simulink model "node23_case_10kV_withLoad_v2"  (R2022b)
settings: Solver=VariableStepAuto  StartTime=0.0  StopTime=10  FixedStep=1e-6  RelTol=1e-5
InitFcn:
  | sw=5;
  | Lf=1.75e-3+3.5e-3;
  | %Lf=3.5e-3;
  | %Cf=2e-4;
  | f=10;
  | Cf=15e-6;
  | % L=1.75e-3/2;
  | % X=100*pi*L;
  | % R=2*X;
  | R=0.25;X=R/0.66;
  | L=X/100/pi;
  | Z=sqrt(R^2+X^2);
  | f = 30;
  | kp1=10;
  | ki1=100;
  | kp4=20;
  | ki4=100;
  | kp16=20;
  | ki16=100;
  | % 负载参数
  | R1L=0;
  | X1L=0;
  | R2L=652.4467;
  | X2L=276.0351;
  | R3L=804.5741;
  | X3L=256.7790;
  | R4L=760.9867;
  | X4L=234.6376;
  | R5L=818.7384;
  | X5L=266.9799;
  | R6L=671.1329;
  | X6L=170.1801;
  | R7L=883.7621;
  | X7L=178.8663;
  | R8L=388.3725;
  | X8L=158.3040;
  | R9L=817.4819;
  | X9L=268.6933;
  | R10L=849.4733;
  | X10L=254.8420;
  | R11L=407.8415;
  | X11L=165.8504;
  | R12L=NaN;  % Bus 12 无 R、X 数据，用 NaN 标记
  | X12L=NaN;
  | R13L=751.2339;
  | X13L=329.8428;
  | R14L=294.0393;
  | X14L=141.6929;
  | R15L=761.9027;
  | X15L=284.3908;
  | R16L=740.4040;
  | X16L=318.2438;
  | R17L=674.5784;
  | X17L=316.4689;
  | R18L=776.7449;
  | X18L=316.6080;
  | R19L=766.0423;
  | X19L=335.7994;
  | R20L=746.0545;
  | X20L=344.3329;
  | ... (+266 lines)
libraries: spsSeriesRLCBranchLib x210, slpidlib x45, spsControlledVoltageSourceLib x30, spsThreePhaseVIMeasurementLib x24, spsPower3phInstantaneousLib x13, spsAlphaBetaZerotoabcLib x9, spsCurrentMeasurementLib x6, spsGroundLib x2, spspowerguiLib x1
(part 7 of 8)

== system node23_case_10kV_withLoad_v2/IBR-23/SOGI ==
  u : Inport
  Gain1 : Gain  Gain=314.15926
  Gain2 : Gain  Gain=0.707
  Gain3 : Gain  Gain=314.15926
  Integrator : Integrator
  Integrator1 : Integrator
  Sum : Sum  Inputs=-+|
  Sum1 : Sum  Inputs=|+-
  u' : Outport
  qu' : Outport  Port=2
  wires:
  Sum/1 -> Gain2/1
  Gain3/1 -> Sum1/2, qu'/1  "qu'"
  Integrator1/1 -> Gain3/1
  Gain2/1 -> Sum1/1
  Integrator/1 -> Sum/1, u'/1, Integrator1/1  "u'"
  u/1 -> Sum/2
  Sum1/1 -> Gain1/1
  Gain1/1 -> Integrator/1

== system node23_case_10kV_withLoad_v2/IBR-23/k=0.3 ==
  u : Inport
  Gain1 : Gain  Gain=314.15926
  Gain2 : Gain  Gain=0.707
  Gain3 : Gain  Gain=314.15926
  Integrator : Integrator
  Integrator1 : Integrator
  Sum : Sum  Inputs=-+|
  Sum1 : Sum  Inputs=|+-
  u' : Outport
  qu' : Outport  Port=2
  wires:
  Sum/1 -> Gain2/1
  Gain3/1 -> Sum1/2, qu'/1  "qu'"
  Integrator1/1 -> Gain3/1
  Gain2/1 -> Sum1/1
  Integrator/1 -> Sum/1, u'/1, Integrator1/1  "u'"
  u/1 -> Sum/2
  Sum1/1 -> Gain1/1
  Gain1/1 -> Integrator/1

== system node23_case_10kV_withLoad_v2/IBR-8/IBR1输出电压正负序分离 ==
  In1 : Inport
  Add1 : Sum  Inputs=+-
  Add2 : Sum
  Add3 : Sum
  Add4 : Sum  Inputs=+-
  Demux2 : Demux  Outputs=3
  Gain{,1..3} (4 alike) : Gain  Gain=0.5
  Gain4 : Gain  Gain=-1
  abc-alphabeta 1 : MATLAB Function  TreatAsAtomicUnit=on
  albe-dq : MATLAB Function  TreatAsAtomicUnit=on
  alphabeta-dq 1 : MATLAB Function  TreatAsAtomicUnit=on
  k=0.1 : Subsystem
  k=0.4 : Subsystem
  Out1 : Outport  VectorParamsAs1DForOutWhenUnconnected=off
  Out2 : Outport  Port=2  VectorParamsAs1DForOutWhenUnconnected=off
  Out3 : Outport  Port=3  VectorParamsAs1DForOutWhenUnconnected=off
  Out4 : Outport  Port=4  VectorParamsAs1DForOutWhenUnconnected=off
  wires:
  Demux2/2 -> abc-alphabeta 1/2(vb)
  k=0.4/1(u') -> Add3/1, Add1/1
  k=0.1/1(u') -> Add4/1, Add2/2
  Add1/1 -> Gain/1
  Demux2/1 -> abc-alphabeta 1/1(va)
  Gain/1 -> alphabeta-dq 1/1(valpha)
  k=0.4/2(qu') -> Add2/1, Add4/2
  albe-dq/1(vd) -> Out3/1
  k=0.1/2(qu') -> Add1/2, Add3/2
  Add2/1 -> Gain1/1
  alphabeta-dq 1/1(vd) -> Out1/1
  Add3/1 -> Gain2/1
  [wt8] -> Gain4/1
  Gain1/1 -> alphabeta-dq 1/2(vbeta)
  In1/1 -> Demux2/1
  Gain2/1 -> albe-dq/1(valpha)
  alphabeta-dq 1/2(vq) -> Out2/1
  Demux2/3 -> abc-alphabeta 1/3(vc)
  [wt8] -> alphabeta-dq 1/3(ph)
  Gain4/1 -> albe-dq/3(ph)
  albe-dq/2(vq) -> Out4/1
  Add4/1 -> Gain3/1
  abc-alphabeta 1/2(vbeta) -> k=0.1/1(u)
  Gain3/1 -> albe-dq/2(vbeta)
  abc-alphabeta 1/1(valpha) -> k=0.4/1(u)

== system node23_case_10kV_withLoad_v2/IBR-8/IBR1输出电流正负序分离 ==
  In1 : Inport
  Add1 : Sum  Inputs=+-
  Add2 : Sum
  Add3 : Sum
  Add4 : Sum  Inputs=+-
  Demux2 : Demux  Outputs=3
  Gain{,1..3} (4 alike) : Gain  Gain=0.5
  Gain4 : Gain  Gain=-1
  abc-alphabeta 1 : MATLAB Function  TreatAsAtomicUnit=on
  albe-dq : MATLAB Function  TreatAsAtomicUnit=on
  alphabeta-dq 1 : MATLAB Function  TreatAsAtomicUnit=on
  k=0.1 : Subsystem
  k=0.4 : Subsystem
  d+ : Outport  VectorParamsAs1DForOutWhenUnconnected=off
  q+ : Outport  Port=2  VectorParamsAs1DForOutWhenUnconnected=off
  d- : Outport  Port=3  VectorParamsAs1DForOutWhenUnconnected=off
  q- : Outport  Port=4  VectorParamsAs1DForOutWhenUnconnected=off
  wires:
  albe-dq/2(vq) -> q-/1
  albe-dq/1(vd) -> d-/1
  alphabeta-dq 1/2(vq) -> q+/1
  alphabeta-dq 1/1(vd) -> d+/1
  abc-alphabeta 1/1(valpha) -> k=0.4/1(u)
  Gain3/1 -> albe-dq/2(vbeta)
  abc-alphabeta 1/2(vbeta) -> k=0.1/1(u)
  Add4/1 -> Gain3/1
  Gain4/1 -> albe-dq/3(ph)
  [wt8] -> alphabeta-dq 1/3(ph)
  Demux2/3 -> abc-alphabeta 1/3(vc)
  Gain2/1 -> albe-dq/1(valpha)
  In1/1 -> Demux2/1
  Gain1/1 -> alphabeta-dq 1/2(vbeta)
  [wt8] -> Gain4/1
  Add3/1 -> Gain2/1
  Add2/1 -> Gain1/1
  k=0.1/2(qu') -> Add3/2, Add1/2
  k=0.4/2(qu') -> Add4/2, Add2/1
  Gain/1 -> alphabeta-dq 1/1(valpha)
  Demux2/1 -> abc-alphabeta 1/1(va)
  Add1/1 -> Gain/1
  k=0.1/1(u') -> Add2/2, Add4/1
  k=0.4/1(u') -> Add1/1, Add3/1
  Demux2/2 -> abc-alphabeta 1/2(vb)

== system node23_case_10kV_withLoad_v2/IBR-8/SOGI ==
  u : Inport
  Gain1 : Gain  Gain=314.15926
  Gain2 : Gain  Gain=0.707
  Gain3 : Gain  Gain=314.15926
  Integrator : Integrator
  Integrator1 : Integrator
  Sum : Sum  Inputs=-+|
  Sum1 : Sum  Inputs=|+-
  u' : Outport
  qu' : Outport  Port=2
  wires:
  Sum/1 -> Gain2/1
  Gain3/1 -> Sum1/2, qu'/1  "qu'"
  Integrator1/1 -> Gain3/1
  Gain2/1 -> Sum1/1
  Integrator/1 -> Sum/1, u'/1, Integrator1/1  "u'"
  u/1 -> Sum/2
  Sum1/1 -> Gain1/1
  Gain1/1 -> Integrator/1

== system node23_case_10kV_withLoad_v2/IBR-8/k=0.3 ==
  u : Inport
  Gain1 : Gain  Gain=314.15926
  Gain2 : Gain  Gain=0.707
  Gain3 : Gain  Gain=314.15926
  Integrator : Integrator
  Integrator1 : Integrator
  Sum : Sum  Inputs=-+|
  Sum1 : Sum  Inputs=|+-
  u' : Outport
  qu' : Outport  Port=2
  wires:
  Sum/1 -> Gain2/1
  Gain3/1 -> Sum1/2, qu'/1  "qu'"
  Integrator1/1 -> Gain3/1
  Gain2/1 -> Sum1/1
  Integrator/1 -> Sum/1, u'/1, Integrator1/1  "u'"
  u/1 -> Sum/2
  Sum1/1 -> Gain1/1
  Gain1/1 -> Integrator/1

== system node23_case_10kV_withLoad_v2/IBR1输出电压正负序分离/k=0.1 ==
  u : Inport
  Gain1 : Gain  Gain=314.15926
  Gain2 : Gain  Gain=0.707
  Gain3 : Gain  Gain=314.15926
  Integrator : Integrator
  Integrator1 : Integrator
  Sum : Sum  Inputs=-+|
  Sum1 : Sum  Inputs=|+-
  u' : Outport
  qu' : Outport  Port=2
  wires:
  Gain1/1 -> Integrator/1
  Sum1/1 -> Gain1/1
  u/1 -> Sum/2
  Integrator/1 -> Integrator1/1, u'/1, Sum/1  "u'"
  Gain2/1 -> Sum1/1
  Integrator1/1 -> Gain3/1
  Gain3/1 -> qu'/1, Sum1/2  "qu'"
  Sum/1 -> Gain2/1

== system node23_case_10kV_withLoad_v2/IBR1输出电压正负序分离/k=0.4 ==
  u : Inport
  Gain1 : Gain  Gain=314.15926
  Gain2 : Gain  Gain=0.707
  Gain3 : Gain  Gain=314.15926
  Integrator : Integrator
  Integrator1 : Integrator
  Sum : Sum  Inputs=-+|
  Sum1 : Sum  Inputs=|+-
  u' : Outport
  qu' : Outport  Port=2
  wires:
  Gain1/1 -> Integrator/1
  Sum1/1 -> Gain1/1
  u/1 -> Sum/2
  Integrator/1 -> Integrator1/1, u'/1, Sum/1  "u'"
  Gain2/1 -> Sum1/1
  Integrator1/1 -> Gain3/1
  Gain3/1 -> qu'/1, Sum1/2  "qu'"
  Sum/1 -> Gain2/1

== system node23_case_10kV_withLoad_v2/IBR1输出电压正负序分离1/k=0.1 ==
  u : Inport
  Gain1 : Gain  Gain=314.15926
  Gain2 : Gain  Gain=0.707
  Gain3 : Gain  Gain=314.15926
  Integrator : Integrator
  Integrator1 : Integrator
  Sum : Sum  Inputs=-+|
  Sum1 : Sum  Inputs=|+-
  u' : Outport
  qu' : Outport  Port=2
  wires:
  Sum/1 -> Gain2/1
  Gain3/1 -> Sum1/2, qu'/1  "qu'"
  Integrator1/1 -> Gain3/1
  Gain2/1 -> Sum1/1
  Integrator/1 -> Sum/1, u'/1, Integrator1/1  "u'"
  u/1 -> Sum/2
  Sum1/1 -> Gain1/1
  Gain1/1 -> Integrator/1

== system node23_case_10kV_withLoad_v2/IBR1输出电压正负序分离1/k=0.4 ==
  u : Inport
  Gain1 : Gain  Gain=314.15926
  Gain2 : Gain  Gain=0.707
  Gain3 : Gain  Gain=314.15926
  Integrator : Integrator
  Integrator1 : Integrator
  Sum : Sum  Inputs=-+|
  Sum1 : Sum  Inputs=|+-
  u' : Outport
  qu' : Outport  Port=2
  wires:
  Sum/1 -> Gain2/1
  Gain3/1 -> Sum1/2, qu'/1  "qu'"
  Integrator1/1 -> Gain3/1
  Gain2/1 -> Sum1/1
  Integrator/1 -> Sum/1, u'/1, Integrator1/1  "u'"
  u/1 -> Sum/2
  Sum1/1 -> Gain1/1
  Gain1/1 -> Integrator/1

== system node23_case_10kV_withLoad_v2/IBR4/IBR1输出电压正负序分离 ==
  In1 : Inport
  Add1 : Sum  Inputs=+-
  Add2 : Sum
  Add3 : Sum
  Add4 : Sum  Inputs=+-
  Demux2 : Demux  Outputs=3
  Gain{,1..3} (4 alike) : Gain  Gain=0.5
  Gain4 : Gain  Gain=-1
  abc-alphabeta 1 : MATLAB Function  TreatAsAtomicUnit=on
  albe-dq : MATLAB Function  TreatAsAtomicUnit=on
  alphabeta-dq 1 : MATLAB Function  TreatAsAtomicUnit=on
  k=0.1 : Subsystem
  k=0.4 : Subsystem
  vcd_p : Outport  VectorParamsAs1DForOutWhenUnconnected=off
  vcq_p : Outport  Port=2  VectorParamsAs1DForOutWhenUnconnected=off
  vcd_n : Outport  Port=3  VectorParamsAs1DForOutWhenUnconnected=off
  vcq_n : Outport  Port=4  VectorParamsAs1DForOutWhenUnconnected=off
  wires:
  abc-alphabeta 1/1(valpha) -> k=0.4/1(u)
  Gain3/1 -> albe-dq/2(vbeta)
  abc-alphabeta 1/2(vbeta) -> k=0.1/1(u)
  Add4/1 -> Gain3/1
  albe-dq/2(vq) -> vcq_n/1
  Gain4/1 -> albe-dq/3(ph)
  [wt4] -> alphabeta-dq 1/3(ph)
  Demux2/3 -> abc-alphabeta 1/3(vc)
  alphabeta-dq 1/2(vq) -> vcq_p/1
  Gain2/1 -> albe-dq/1(valpha)
  In1/1 -> Demux2/1
  Gain1/1 -> alphabeta-dq 1/2(vbeta)
  [wt4] -> Gain4/1
  Add3/1 -> Gain2/1
  alphabeta-dq 1/1(vd) -> vcd_p/1
  Add2/1 -> Gain1/1
  k=0.1/2(qu') -> Add3/2, Add1/2
  albe-dq/1(vd) -> vcd_n/1
  k=0.4/2(qu') -> Add4/2, Add2/1
  Gain/1 -> alphabeta-dq 1/1(valpha)
  Demux2/1 -> abc-alphabeta 1/1(va)
  Add1/1 -> Gain/1
  k=0.1/1(u') -> Add2/2, Add4/1
  k=0.4/1(u') -> Add1/1, Add3/1
  Demux2/2 -> abc-alphabeta 1/2(vb)

== system node23_case_10kV_withLoad_v2/IBR4/IBR1输出电流正负序分离 ==
  In1 : Inport
  Add1 : Sum  Inputs=+-
  Add2 : Sum
  Add3 : Sum
  Add4 : Sum  Inputs=+-
  Demux2 : Demux  Outputs=3
  Gain{,1..3} (4 alike) : Gain  Gain=0.5
  Gain4 : Gain  Gain=-1
  abc-alphabeta 1 : MATLAB Function  TreatAsAtomicUnit=on
  albe-dq : MATLAB Function  TreatAsAtomicUnit=on
  alphabeta-dq 1 : MATLAB Function  TreatAsAtomicUnit=on
  k=0.1 : Subsystem
  k=0.4 : Subsystem
  d+ : Outport  VectorParamsAs1DForOutWhenUnconnected=off
  q+ : Outport  Port=2  VectorParamsAs1DForOutWhenUnconnected=off
  d- : Outport  Port=3  VectorParamsAs1DForOutWhenUnconnected=off
  q- : Outport  Port=4  VectorParamsAs1DForOutWhenUnconnected=off
  wires:
  Demux2/2 -> abc-alphabeta 1/2(vb)
  k=0.4/1(u') -> Add3/1, Add1/1
  k=0.1/1(u') -> Add4/1, Add2/2
  Add1/1 -> Gain/1
  Demux2/1 -> abc-alphabeta 1/1(va)
  Gain/1 -> alphabeta-dq 1/1(valpha)
  k=0.4/2(qu') -> Add2/1, Add4/2
  k=0.1/2(qu') -> Add1/2, Add3/2
  Add2/1 -> Gain1/1
  Add3/1 -> Gain2/1
  [wt4] -> Gain4/1
  Gain1/1 -> alphabeta-dq 1/2(vbeta)
  In1/1 -> Demux2/1
  Gain2/1 -> albe-dq/1(valpha)
  Demux2/3 -> abc-alphabeta 1/3(vc)
  [wt4] -> alphabeta-dq 1/3(ph)
  Gain4/1 -> albe-dq/3(ph)
  Add4/1 -> Gain3/1
  abc-alphabeta 1/2(vbeta) -> k=0.1/1(u)
  Gain3/1 -> albe-dq/2(vbeta)
  abc-alphabeta 1/1(valpha) -> k=0.4/1(u)
  alphabeta-dq 1/1(vd) -> d+/1
  alphabeta-dq 1/2(vq) -> q+/1
  albe-dq/1(vd) -> d-/1
  albe-dq/2(vq) -> q-/1

== system node23_case_10kV_withLoad_v2/IBR4/SOGI ==
  u : Inport
  Gain1 : Gain  Gain=314.15926
  Gain2 : Gain  Gain=0.707
  Gain3 : Gain  Gain=314.15926
  Integrator : Integrator
  Integrator1 : Integrator
  Sum : Sum  Inputs=-+|
  Sum1 : Sum  Inputs=|+-
  u' : Outport
  qu' : Outport  Port=2
  wires:
  Sum/1 -> Gain2/1
  Gain3/1 -> Sum1/2, qu'/1  "qu'"
  Integrator1/1 -> Gain3/1
  Gain2/1 -> Sum1/1
  Integrator/1 -> Sum/1, u'/1, Integrator1/1  "u'"
  u/1 -> Sum/2
  Sum1/1 -> Gain1/1
  Gain1/1 -> Integrator/1

== system node23_case_10kV_withLoad_v2/IBR4/k=0.3 ==
  u : Inport
  Gain1 : Gain  Gain=314.15926
  Gain2 : Gain  Gain=0.707
  Gain3 : Gain  Gain=314.15926
  Integrator : Integrator
  Integrator1 : Integrator
  Sum : Sum  Inputs=-+|
  Sum1 : Sum  Inputs=|+-
  u' : Outport
  qu' : Outport  Port=2
  wires:
  Sum/1 -> Gain2/1
  Gain3/1 -> Sum1/2, qu'/1  "qu'"
  Integrator1/1 -> Gain3/1
  Gain2/1 -> Sum1/1
  Integrator/1 -> Sum/1, u'/1, Integrator1/1  "u'"
  u/1 -> Sum/2
  Sum1/1 -> Gain1/1
  Gain1/1 -> Integrator/1

== system node23_case_10kV_withLoad_v2/电网电压正负序分离/k=0.1 ==
  u : Inport
  Gain1 : Gain  Gain=314.15926
  Gain2 : Gain  Gain=0.707
  Gain3 : Gain  Gain=314.15926
  Integrator : Integrator
  Integrator1 : Integrator
  Sum : Sum  Inputs=-+|
  Sum1 : Sum  Inputs=|+-
  u' : Outport
  qu' : Outport  Port=2
  wires:
  Gain1/1 -> Integrator/1
  Sum1/1 -> Gain1/1
  u/1 -> Sum/2
  Integrator/1 -> Integrator1/1, u'/1, Sum/1  "u'"
  Gain2/1 -> Sum1/1
  Integrator1/1 -> Gain3/1
  Gain3/1 -> qu'/1, Sum1/2  "qu'"
  Sum/1 -> Gain2/1

== system node23_case_10kV_withLoad_v2/电网电压正负序分离/k=0.4 ==
  u : Inport
  Gain1 : Gain  Gain=314.15926
  Gain2 : Gain  Gain=0.707
  Gain3 : Gain  Gain=314.15926
  Integrator : Integrator
  Integrator1 : Integrator
  Sum : Sum  Inputs=-+|
  Sum1 : Sum  Inputs=|+-
  u' : Outport
  qu' : Outport  Port=2
  wires:
  Gain1/1 -> Integrator/1
  Sum1/1 -> Gain1/1
  u/1 -> Sum/2
  Integrator/1 -> Integrator1/1, u'/1, Sum/1  "u'"
  Gain2/1 -> Sum1/1
  Integrator1/1 -> Gain3/1
  Gain3/1 -> qu'/1, Sum1/2  "qu'"
  Sum/1 -> Gain2/1

== system node23_case_10kV_withLoad_v2/Grid/negative_sequence_dq>>abc4/dq0>>alpha_beta_0 ==
  alpha_beta_0 : Inport
  Gain3 : Gain  Gain="[ 1   0   1; -1/2  sqrt(3)/2   1; -1/2  -sqrt(3)/2  1 ]"  Multiplication=Matrix(K*u) (u vector)  SaturateOnIntegerOverflow=on  OutDataTypeStr=Inherit: Same as input  ParamDataTypeStr=Inherit: Same as input
  abc : Outport
  wires:
  alpha_beta_0/1 -> Gain3/1
  Gain3/1 -> abc/1

== system node23_case_10kV_withLoad_v2/Grid/positive_sequence_dq>>abc1/dq0>>alpha_beta_0 ==
  alpha_beta_0 : Inport
  Gain3 : Gain  Gain="[ 1   0   1; -1/2  sqrt(3)/2   1; -1/2  -sqrt(3)/2  1 ]"  Multiplication=Matrix(K*u) (u vector)  SaturateOnIntegerOverflow=on  OutDataTypeStr=Inherit: Same as input  ParamDataTypeStr=Inherit: Same as input
  abc : Outport
  wires:
  alpha_beta_0/1 -> Gain3/1
  Gain3/1 -> abc/1

== system node23_case_10kV_withLoad_v2/IBR-10/IBR1输出电压正负序分离/k=0.1 ==
  u : Inport
  Gain1 : Gain  Gain=314.15926
  Gain2 : Gain  Gain=0.707
  Gain3 : Gain  Gain=314.15926
  Integrator : Integrator
  Integrator1 : Integrator
  Sum : Sum  Inputs=-+|
  Sum1 : Sum  Inputs=|+-
  u' : Outport
  qu' : Outport  Port=2
  wires:
  Sum/1 -> Gain2/1
  Gain3/1 -> Sum1/2, qu'/1  "qu'"
  Integrator1/1 -> Gain3/1
  Gain2/1 -> Sum1/1
  Integrator/1 -> Sum/1, u'/1, Integrator1/1  "u'"
  u/1 -> Sum/2
  Sum1/1 -> Gain1/1
  Gain1/1 -> Integrator/1

== system node23_case_10kV_withLoad_v2/IBR-10/IBR1输出电压正负序分离/k=0.4 ==
  u : Inport
  Gain1 : Gain  Gain=314.15926
  Gain2 : Gain  Gain=0.707
  Gain3 : Gain  Gain=314.15926
  Integrator : Integrator
  Integrator1 : Integrator
  Sum : Sum  Inputs=-+|
  Sum1 : Sum  Inputs=|+-
  u' : Outport
  qu' : Outport  Port=2
  wires:
  Sum/1 -> Gain2/1
  Gain3/1 -> Sum1/2, qu'/1  "qu'"
  Integrator1/1 -> Gain3/1
  Gain2/1 -> Sum1/1
  Integrator/1 -> Sum/1, u'/1, Integrator1/1  "u'"
  u/1 -> Sum/2
  Sum1/1 -> Gain1/1
  Gain1/1 -> Integrator/1

== system node23_case_10kV_withLoad_v2/IBR-10/IBR1输出电流正负序分离/k=0.1 ==
  u : Inport
  Gain1 : Gain  Gain=314.15926
  Gain2 : Gain  Gain=0.707
  Gain3 : Gain  Gain=314.15926
  Integrator : Integrator
  Integrator1 : Integrator
  Sum : Sum  Inputs=-+|
  Sum1 : Sum  Inputs=|+-
  u' : Outport
  qu' : Outport  Port=2
  wires:
  Gain1/1 -> Integrator/1
  Sum1/1 -> Gain1/1
  u/1 -> Sum/2
  Integrator/1 -> Integrator1/1, u'/1, Sum/1  "u'"
  Gain2/1 -> Sum1/1
  Integrator1/1 -> Gain3/1
  Gain3/1 -> qu'/1, Sum1/2  "qu'"
  Sum/1 -> Gain2/1

== system node23_case_10kV_withLoad_v2/IBR-10/IBR1输出电流正负序分离/k=0.4 ==
  u : Inport
  Gain1 : Gain  Gain=314.15926
  Gain2 : Gain  Gain=0.707
  Gain3 : Gain  Gain=314.15926
  Integrator : Integrator
  Integrator1 : Integrator
  Sum : Sum  Inputs=-+|
  Sum1 : Sum  Inputs=|+-
  u' : Outport
  qu' : Outport  Port=2
  wires:
  Gain1/1 -> Integrator/1
  Sum1/1 -> Gain1/1
  u/1 -> Sum/2
  Integrator/1 -> Integrator1/1, u'/1, Sum/1  "u'"
  Gain2/1 -> Sum1/1
  Integrator1/1 -> Gain3/1
  Gain3/1 -> qu'/1, Sum1/2  "qu'"
  Sum/1 -> Gain2/1

== system node23_case_10kV_withLoad_v2/IBR-11/IBR1输出电压正负序分离/k=0.1 ==
  u : Inport
  Gain1 : Gain  Gain=314.15926
  Gain2 : Gain  Gain=0.707
  Gain3 : Gain  Gain=314.15926
  Integrator : Integrator
  Integrator1 : Integrator
  Sum : Sum  Inputs=-+|
  Sum1 : Sum  Inputs=|+-
  u' : Outport
  qu' : Outport  Port=2
  wires:
  Sum/1 -> Gain2/1
  Gain3/1 -> Sum1/2, qu'/1  "qu'"
  Integrator1/1 -> Gain3/1
  Gain2/1 -> Sum1/1
  Integrator/1 -> Sum/1, u'/1, Integrator1/1  "u'"
  u/1 -> Sum/2
  Sum1/1 -> Gain1/1
  Gain1/1 -> Integrator/1

== system node23_case_10kV_withLoad_v2/IBR-11/IBR1输出电压正负序分离/k=0.4 ==
  u : Inport
  Gain1 : Gain  Gain=314.15926
  Gain2 : Gain  Gain=0.707
  Gain3 : Gain  Gain=314.15926
  Integrator : Integrator
  Integrator1 : Integrator
  Sum : Sum  Inputs=-+|
  Sum1 : Sum  Inputs=|+-
  u' : Outport
  qu' : Outport  Port=2
  wires:
  Sum/1 -> Gain2/1
  Gain3/1 -> Sum1/2, qu'/1  "qu'"
  Integrator1/1 -> Gain3/1
  Gain2/1 -> Sum1/1
  Integrator/1 -> Sum/1, u'/1, Integrator1/1  "u'"
  u/1 -> Sum/2
  Sum1/1 -> Gain1/1
  Gain1/1 -> Integrator/1

== system node23_case_10kV_withLoad_v2/IBR-11/IBR1输出电流正负序分离/k=0.1 ==
  u : Inport
  Gain1 : Gain  Gain=314.15926
  Gain2 : Gain  Gain=0.707
  Gain3 : Gain  Gain=314.15926
  Integrator : Integrator
  Integrator1 : Integrator
  Sum : Sum  Inputs=-+|
  Sum1 : Sum  Inputs=|+-
  u' : Outport
  qu' : Outport  Port=2
  wires:
  Gain1/1 -> Integrator/1
  Sum1/1 -> Gain1/1
  u/1 -> Sum/2
  Integrator/1 -> Integrator1/1, u'/1, Sum/1  "u'"
  Gain2/1 -> Sum1/1
  Integrator1/1 -> Gain3/1
  Gain3/1 -> qu'/1, Sum1/2  "qu'"
  Sum/1 -> Gain2/1

== system node23_case_10kV_withLoad_v2/IBR-11/IBR1输出电流正负序分离/k=0.4 ==
  u : Inport
  Gain1 : Gain  Gain=314.15926
  Gain2 : Gain  Gain=0.707
  Gain3 : Gain  Gain=314.15926
  Integrator : Integrator
  Integrator1 : Integrator
  Sum : Sum  Inputs=-+|
  Sum1 : Sum  Inputs=|+-
  u' : Outport
  qu' : Outport  Port=2
  wires:
  Gain1/1 -> Integrator/1
  Sum1/1 -> Gain1/1
  u/1 -> Sum/2
  Integrator/1 -> Integrator1/1, u'/1, Sum/1  "u'"
  Gain2/1 -> Sum1/1
  Integrator1/1 -> Gain3/1
  Gain3/1 -> qu'/1, Sum1/2  "qu'"
  Sum/1 -> Gain2/1

== system node23_case_10kV_withLoad_v2/IBR-12/IBR1输出电压正负序分离/k=0.1 ==
  u : Inport
  Gain1 : Gain  Gain=314.15926
  Gain2 : Gain  Gain=0.707
  Gain3 : Gain  Gain=314.15926
  Integrator : Integrator
  Integrator1 : Integrator
  Sum : Sum  Inputs=-+|
  Sum1 : Sum  Inputs=|+-
  u' : Outport
  qu' : Outport  Port=2
  wires:
  Sum/1 -> Gain2/1
  Gain3/1 -> Sum1/2, qu'/1  "qu'"
  Integrator1/1 -> Gain3/1
  Gain2/1 -> Sum1/1
  Integrator/1 -> Sum/1, u'/1, Integrator1/1  "u'"
  u/1 -> Sum/2
  Sum1/1 -> Gain1/1
  Gain1/1 -> Integrator/1

== system node23_case_10kV_withLoad_v2/IBR-12/IBR1输出电压正负序分离/k=0.4 ==
  u : Inport
  Gain1 : Gain  Gain=314.15926
  Gain2 : Gain  Gain=0.707
  Gain3 : Gain  Gain=314.15926
  Integrator : Integrator
  Integrator1 : Integrator
  Sum : Sum  Inputs=-+|
  Sum1 : Sum  Inputs=|+-
  u' : Outport
  qu' : Outport  Port=2
  wires:
  Sum/1 -> Gain2/1
  Gain3/1 -> Sum1/2, qu'/1  "qu'"
  Integrator1/1 -> Gain3/1
  Gain2/1 -> Sum1/1
  Integrator/1 -> Sum/1, u'/1, Integrator1/1  "u'"
  u/1 -> Sum/2
  Sum1/1 -> Gain1/1
  Gain1/1 -> Integrator/1

== system node23_case_10kV_withLoad_v2/IBR-12/IBR1输出电流正负序分离/k=0.1 ==
  u : Inport
  Gain1 : Gain  Gain=314.15926
  Gain2 : Gain  Gain=0.707
  Gain3 : Gain  Gain=314.15926
  Integrator : Integrator
  Integrator1 : Integrator
  Sum : Sum  Inputs=-+|
  Sum1 : Sum  Inputs=|+-
  u' : Outport
  qu' : Outport  Port=2
  wires:
  Gain1/1 -> Integrator/1
  Sum1/1 -> Gain1/1
  u/1 -> Sum/2
  Integrator/1 -> Integrator1/1, u'/1, Sum/1  "u'"
  Gain2/1 -> Sum1/1
  Integrator1/1 -> Gain3/1
  Gain3/1 -> qu'/1, Sum1/2  "qu'"
  Sum/1 -> Gain2/1

== system node23_case_10kV_withLoad_v2/IBR-12/IBR1输出电流正负序分离/k=0.4 ==
  u : Inport
  Gain1 : Gain  Gain=314.15926
  Gain2 : Gain  Gain=0.707
  Gain3 : Gain  Gain=314.15926
  Integrator : Integrator
  Integrator1 : Integrator
  Sum : Sum  Inputs=-+|
  Sum1 : Sum  Inputs=|+-
  u' : Outport
  qu' : Outport  Port=2
  wires:
  Gain1/1 -> Integrator/1
  Sum1/1 -> Gain1/1
  u/1 -> Sum/2
  Integrator/1 -> Integrator1/1, u'/1, Sum/1  "u'"
  Gain2/1 -> Sum1/1
  Integrator1/1 -> Gain3/1
  Gain3/1 -> qu'/1, Sum1/2  "qu'"
  Sum/1 -> Gain2/1

== system node23_case_10kV_withLoad_v2/IBR-16/IBR1输出电压正负序分离/k=0.1 ==
  u : Inport
  Gain1 : Gain  Gain=314.15926
  Gain2 : Gain  Gain=0.707
  Gain3 : Gain  Gain=314.15926
  Integrator : Integrator
  Integrator1 : Integrator
  Sum : Sum  Inputs=-+|
  Sum1 : Sum  Inputs=|+-
  u' : Outport
  qu' : Outport  Port=2
  wires:
  Sum/1 -> Gain2/1
  Gain3/1 -> Sum1/2, qu'/1  "qu'"
  Integrator1/1 -> Gain3/1
  Gain2/1 -> Sum1/1
  Integrator/1 -> Sum/1, u'/1, Integrator1/1  "u'"
  u/1 -> Sum/2
  Sum1/1 -> Gain1/1
  Gain1/1 -> Integrator/1

== system node23_case_10kV_withLoad_v2/IBR-16/IBR1输出电压正负序分离/k=0.4 ==
  u : Inport
  Gain1 : Gain  Gain=314.15926
  Gain2 : Gain  Gain=0.707
  Gain3 : Gain  Gain=314.15926
  Integrator : Integrator
  Integrator1 : Integrator
  Sum : Sum  Inputs=-+|
  Sum1 : Sum  Inputs=|+-
  u' : Outport
  qu' : Outport  Port=2
  wires:
  Sum/1 -> Gain2/1
  Gain3/1 -> Sum1/2, qu'/1  "qu'"
  Integrator1/1 -> Gain3/1
  Gain2/1 -> Sum1/1
  Integrator/1 -> Sum/1, u'/1, Integrator1/1  "u'"
  u/1 -> Sum/2
  Sum1/1 -> Gain1/1
  Gain1/1 -> Integrator/1

== system node23_case_10kV_withLoad_v2/IBR-16/IBR1输出电流正负序分离/k=0.1 ==
  u : Inport
  Gain1 : Gain  Gain=314.15926
  Gain2 : Gain  Gain=0.707
  Gain3 : Gain  Gain=314.15926
  Integrator : Integrator
  Integrator1 : Integrator
  Sum : Sum  Inputs=-+|
  Sum1 : Sum  Inputs=|+-
  u' : Outport
  qu' : Outport  Port=2
  wires:
  Gain1/1 -> Integrator/1
  Sum1/1 -> Gain1/1
  u/1 -> Sum/2
  Integrator/1 -> Integrator1/1, u'/1, Sum/1  "u'"
  Gain2/1 -> Sum1/1
  Integrator1/1 -> Gain3/1
  Gain3/1 -> qu'/1, Sum1/2  "qu'"
  Sum/1 -> Gain2/1

== system node23_case_10kV_withLoad_v2/IBR-16/IBR1输出电流正负序分离/k=0.4 ==
  u : Inport
  Gain1 : Gain  Gain=314.15926
  Gain2 : Gain  Gain=0.707
  Gain3 : Gain  Gain=314.15926
  Integrator : Integrator
  Integrator1 : Integrator
  Sum : Sum  Inputs=-+|
  Sum1 : Sum  Inputs=|+-
  u' : Outport
  qu' : Outport  Port=2
  wires:
  Gain1/1 -> Integrator/1
  Sum1/1 -> Gain1/1
  u/1 -> Sum/2
  Integrator/1 -> Integrator1/1, u'/1, Sum/1  "u'"
  Gain2/1 -> Sum1/1
  Integrator1/1 -> Gain3/1
  Gain3/1 -> qu'/1, Sum1/2  "qu'"
  Sum/1 -> Gain2/1

== system node23_case_10kV_withLoad_v2/IBR-21/IBR1输出电压正负序分离/k=0.1 ==
  u : Inport
  Gain1 : Gain  Gain=314.15926
  Gain2 : Gain  Gain=0.707
  Gain3 : Gain  Gain=314.15926
  Integrator : Integrator
  Integrator1 : Integrator
  Sum : Sum  Inputs=-+|
  Sum1 : Sum  Inputs=|+-
  u' : Outport
  qu' : Outport  Port=2
  wires:
  Sum/1 -> Gain2/1
  Gain3/1 -> Sum1/2, qu'/1  "qu'"
  Integrator1/1 -> Gain3/1
  Gain2/1 -> Sum1/1
  Integrator/1 -> Sum/1, u'/1, Integrator1/1  "u'"
  u/1 -> Sum/2
  Sum1/1 -> Gain1/1
  Gain1/1 -> Integrator/1

== system node23_case_10kV_withLoad_v2/IBR-21/IBR1输出电压正负序分离/k=0.4 ==
  u : Inport
  Gain1 : Gain  Gain=314.15926
  Gain2 : Gain  Gain=0.707
  Gain3 : Gain  Gain=314.15926
  Integrator : Integrator
  Integrator1 : Integrator
  Sum : Sum  Inputs=-+|
  Sum1 : Sum  Inputs=|+-
  u' : Outport
  qu' : Outport  Port=2
  wires:
  Sum/1 -> Gain2/1
  Gain3/1 -> Sum1/2, qu'/1  "qu'"
  Integrator1/1 -> Gain3/1
  Gain2/1 -> Sum1/1
  Integrator/1 -> Sum/1, u'/1, Integrator1/1  "u'"
  u/1 -> Sum/2
  Sum1/1 -> Gain1/1
  Gain1/1 -> Integrator/1

== system node23_case_10kV_withLoad_v2/IBR-21/IBR1输出电流正负序分离/k=0.1 ==
  u : Inport
  Gain1 : Gain  Gain=314.15926
  Gain2 : Gain  Gain=0.707
  Gain3 : Gain  Gain=314.15926
  Integrator : Integrator
  Integrator1 : Integrator
  Sum : Sum  Inputs=-+|
  Sum1 : Sum  Inputs=|+-
  u' : Outport
  qu' : Outport  Port=2
  wires:
  Gain1/1 -> Integrator/1
  Sum1/1 -> Gain1/1
  u/1 -> Sum/2
  Integrator/1 -> Integrator1/1, u'/1, Sum/1  "u'"
  Gain2/1 -> Sum1/1
  Integrator1/1 -> Gain3/1
  Gain3/1 -> qu'/1, Sum1/2  "qu'"
  Sum/1 -> Gain2/1

== system node23_case_10kV_withLoad_v2/IBR-21/IBR1输出电流正负序分离/k=0.4 ==
  u : Inport
  Gain1 : Gain  Gain=314.15926
  Gain2 : Gain  Gain=0.707
  Gain3 : Gain  Gain=314.15926
  Integrator : Integrator
  Integrator1 : Integrator
  Sum : Sum  Inputs=-+|
  Sum1 : Sum  Inputs=|+-
  u' : Outport
  qu' : Outport  Port=2
  wires:
  Gain1/1 -> Integrator/1
  Sum1/1 -> Gain1/1
  u/1 -> Sum/2
  Integrator/1 -> Integrator1/1, u'/1, Sum/1  "u'"
  Gain2/1 -> Sum1/1
  Integrator1/1 -> Gain3/1
  Gain3/1 -> qu'/1, Sum1/2  "qu'"
  Sum/1 -> Gain2/1

== system node23_case_10kV_withLoad_v2/IBR-22/IBR1输出电压正负序分离/k=0.1 ==
  u : Inport
  Gain1 : Gain  Gain=314.15926
  Gain2 : Gain  Gain=0.707
  Gain3 : Gain  Gain=314.15926
  Integrator : Integrator
  Integrator1 : Integrator
  Sum : Sum  Inputs=-+|
  Sum1 : Sum  Inputs=|+-
  u' : Outport
  qu' : Outport  Port=2
  wires:
  Sum/1 -> Gain2/1
  Gain3/1 -> Sum1/2, qu'/1  "qu'"
  Integrator1/1 -> Gain3/1
  Gain2/1 -> Sum1/1
  Integrator/1 -> Sum/1, u'/1, Integrator1/1  "u'"
  u/1 -> Sum/2
  Sum1/1 -> Gain1/1
  Gain1/1 -> Integrator/1

== system node23_case_10kV_withLoad_v2/IBR-22/IBR1输出电压正负序分离/k=0.4 ==
  u : Inport
  Gain1 : Gain  Gain=314.15926
  Gain2 : Gain  Gain=0.707
  Gain3 : Gain  Gain=314.15926
  Integrator : Integrator
  Integrator1 : Integrator
  Sum : Sum  Inputs=-+|
  Sum1 : Sum  Inputs=|+-
  u' : Outport
  qu' : Outport  Port=2
  wires:
  Sum/1 -> Gain2/1
  Gain3/1 -> Sum1/2, qu'/1  "qu'"
  Integrator1/1 -> Gain3/1
  Gain2/1 -> Sum1/1
  Integrator/1 -> Sum/1, u'/1, Integrator1/1  "u'"
  u/1 -> Sum/2
  Sum1/1 -> Gain1/1
  Gain1/1 -> Integrator/1

== system node23_case_10kV_withLoad_v2/IBR-22/IBR1输出电流正负序分离/k=0.1 ==
  u : Inport
  Gain1 : Gain  Gain=314.15926
  Gain2 : Gain  Gain=0.707
  Gain3 : Gain  Gain=314.15926
  Integrator : Integrator
  Integrator1 : Integrator
  Sum : Sum  Inputs=-+|
  Sum1 : Sum  Inputs=|+-
  u' : Outport
  qu' : Outport  Port=2
  wires:
  Gain1/1 -> Integrator/1
  Sum1/1 -> Gain1/1
  u/1 -> Sum/2
  Integrator/1 -> Integrator1/1, u'/1, Sum/1  "u'"
  Gain2/1 -> Sum1/1
  Integrator1/1 -> Gain3/1
  Gain3/1 -> qu'/1, Sum1/2  "qu'"
  Sum/1 -> Gain2/1

== system node23_case_10kV_withLoad_v2/IBR-22/IBR1输出电流正负序分离/k=0.4 ==
  u : Inport
  Gain1 : Gain  Gain=314.15926
  Gain2 : Gain  Gain=0.707
  Gain3 : Gain  Gain=314.15926
  Integrator : Integrator
  Integrator1 : Integrator
  Sum : Sum  Inputs=-+|
  Sum1 : Sum  Inputs=|+-
  u' : Outport
  qu' : Outport  Port=2
  wires:
  Gain1/1 -> Integrator/1
  Sum1/1 -> Gain1/1
  u/1 -> Sum/2
  Integrator/1 -> Integrator1/1, u'/1, Sum/1  "u'"
  Gain2/1 -> Sum1/1
  Integrator1/1 -> Gain3/1
  Gain3/1 -> qu'/1, Sum1/2  "qu'"
  Sum/1 -> Gain2/1

== system node23_case_10kV_withLoad_v2/IBR-23/IBR1输出电压正负序分离/k=0.1 ==
  u : Inport
  Gain1 : Gain  Gain=314.15926
  Gain2 : Gain  Gain=0.707
  Gain3 : Gain  Gain=314.15926
  Integrator : Integrator
  Integrator1 : Integrator
  Sum : Sum  Inputs=-+|
  Sum1 : Sum  Inputs=|+-
  u' : Outport
  qu' : Outport  Port=2
  wires:
  Sum/1 -> Gain2/1
  Gain3/1 -> Sum1/2, qu'/1  "qu'"
  Integrator1/1 -> Gain3/1
  Gain2/1 -> Sum1/1
  Integrator/1 -> Sum/1, u'/1, Integrator1/1  "u'"
  u/1 -> Sum/2
  Sum1/1 -> Gain1/1
  Gain1/1 -> Integrator/1

== system node23_case_10kV_withLoad_v2/IBR-23/IBR1输出电压正负序分离/k=0.4 ==
  u : Inport
  Gain1 : Gain  Gain=314.15926
  Gain2 : Gain  Gain=0.707
  Gain3 : Gain  Gain=314.15926
  Integrator : Integrator
  Integrator1 : Integrator
  Sum : Sum  Inputs=-+|
  Sum1 : Sum  Inputs=|+-
  u' : Outport
  qu' : Outport  Port=2
  wires:
  Sum/1 -> Gain2/1
  Gain3/1 -> Sum1/2, qu'/1  "qu'"
  Integrator1/1 -> Gain3/1
  Gain2/1 -> Sum1/1
  Integrator/1 -> Sum/1, u'/1, Integrator1/1  "u'"
  u/1 -> Sum/2
  Sum1/1 -> Gain1/1
  Gain1/1 -> Integrator/1

== system node23_case_10kV_withLoad_v2/IBR-23/IBR1输出电流正负序分离/k=0.1 ==
  u : Inport
  Gain1 : Gain  Gain=314.15926
  Gain2 : Gain  Gain=0.707
  Gain3 : Gain  Gain=314.15926
  Integrator : Integrator
  Integrator1 : Integrator
  Sum : Sum  Inputs=-+|
  Sum1 : Sum  Inputs=|+-
  u' : Outport
  qu' : Outport  Port=2
  wires:
  Gain1/1 -> Integrator/1
  Sum1/1 -> Gain1/1
  u/1 -> Sum/2
  Integrator/1 -> Integrator1/1, u'/1, Sum/1  "u'"
  Gain2/1 -> Sum1/1
  Integrator1/1 -> Gain3/1
  Gain3/1 -> qu'/1, Sum1/2  "qu'"
  Sum/1 -> Gain2/1

== system node23_case_10kV_withLoad_v2/IBR-23/IBR1输出电流正负序分离/k=0.4 ==
  u : Inport
  Gain1 : Gain  Gain=314.15926
  Gain2 : Gain  Gain=0.707
  Gain3 : Gain  Gain=314.15926
  Integrator : Integrator
  Integrator1 : Integrator
  Sum : Sum  Inputs=-+|
  Sum1 : Sum  Inputs=|+-
  u' : Outport
  qu' : Outport  Port=2
  wires:
  Gain1/1 -> Integrator/1
  Sum1/1 -> Gain1/1
  u/1 -> Sum/2
  Integrator/1 -> Integrator1/1, u'/1, Sum/1  "u'"
  Gain2/1 -> Sum1/1
  Integrator1/1 -> Gain3/1
  Gain3/1 -> qu'/1, Sum1/2  "qu'"
  Sum/1 -> Gain2/1

== system node23_case_10kV_withLoad_v2/IBR-8/IBR1输出电压正负序分离/k=0.1 ==
  u : Inport
  Gain1 : Gain  Gain=314.15926
  Gain2 : Gain  Gain=0.707
  Gain3 : Gain  Gain=314.15926
  Integrator : Integrator
  Integrator1 : Integrator
  Sum : Sum  Inputs=-+|
  Sum1 : Sum  Inputs=|+-
  u' : Outport
  qu' : Outport  Port=2
  wires:
  Sum/1 -> Gain2/1
  Gain3/1 -> Sum1/2, qu'/1  "qu'"
  Integrator1/1 -> Gain3/1
  Gain2/1 -> Sum1/1
  Integrator/1 -> Sum/1, u'/1, Integrator1/1  "u'"
  u/1 -> Sum/2
  Sum1/1 -> Gain1/1
  Gain1/1 -> Integrator/1

== system node23_case_10kV_withLoad_v2/IBR-8/IBR1输出电压正负序分离/k=0.4 ==
  u : Inport
  Gain1 : Gain  Gain=314.15926
  Gain2 : Gain  Gain=0.707
  Gain3 : Gain  Gain=314.15926
  Integrator : Integrator
  Integrator1 : Integrator
  Sum : Sum  Inputs=-+|
  Sum1 : Sum  Inputs=|+-
  u' : Outport
  qu' : Outport  Port=2
  wires:
  Sum/1 -> Gain2/1
  Gain3/1 -> Sum1/2, qu'/1  "qu'"
  Integrator1/1 -> Gain3/1
  Gain2/1 -> Sum1/1
  Integrator/1 -> Sum/1, u'/1, Integrator1/1  "u'"
  u/1 -> Sum/2
  Sum1/1 -> Gain1/1
  Gain1/1 -> Integrator/1

== system node23_case_10kV_withLoad_v2/IBR-8/IBR1输出电流正负序分离/k=0.1 ==
  u : Inport
  Gain1 : Gain  Gain=314.15926
  Gain2 : Gain  Gain=0.707
  Gain3 : Gain  Gain=314.15926
  Integrator : Integrator
  Integrator1 : Integrator
  Sum : Sum  Inputs=-+|
  Sum1 : Sum  Inputs=|+-
  u' : Outport
  qu' : Outport  Port=2
  wires:
  Gain1/1 -> Integrator/1
  Sum1/1 -> Gain1/1
  u/1 -> Sum/2
  Integrator/1 -> Integrator1/1, u'/1, Sum/1  "u'"
  Gain2/1 -> Sum1/1
  Integrator1/1 -> Gain3/1
  Gain3/1 -> qu'/1, Sum1/2  "qu'"
  Sum/1 -> Gain2/1

== system node23_case_10kV_withLoad_v2/IBR-8/IBR1输出电流正负序分离/k=0.4 ==
  u : Inport
  Gain1 : Gain  Gain=314.15926
  Gain2 : Gain  Gain=0.707
  Gain3 : Gain  Gain=314.15926
  Integrator : Integrator
  Integrator1 : Integrator
  Sum : Sum  Inputs=-+|
  Sum1 : Sum  Inputs=|+-
  u' : Outport
  qu' : Outport  Port=2
  wires:
  Gain1/1 -> Integrator/1
  Sum1/1 -> Gain1/1
  u/1 -> Sum/2
  Integrator/1 -> Integrator1/1, u'/1, Sum/1  "u'"
  Gain2/1 -> Sum1/1
  Integrator1/1 -> Gain3/1
  Gain3/1 -> qu'/1, Sum1/2  "qu'"
  Sum/1 -> Gain2/1

== system node23_case_10kV_withLoad_v2/IBR4/IBR1输出电压正负序分离/k=0.1 ==
  u : Inport
  Gain1 : Gain  Gain=314.15926
  Gain2 : Gain  Gain=0.707
  Gain3 : Gain  Gain=314.15926
  Integrator : Integrator
  Integrator1 : Integrator
  Sum : Sum  Inputs=-+|
  Sum1 : Sum  Inputs=|+-
  u' : Outport
  qu' : Outport  Port=2
  wires:
  Gain1/1 -> Integrator/1
  Sum1/1 -> Gain1/1
  u/1 -> Sum/2
  Integrator/1 -> Integrator1/1, u'/1, Sum/1  "u'"
  Gain2/1 -> Sum1/1
  Integrator1/1 -> Gain3/1
  Gain3/1 -> qu'/1, Sum1/2  "qu'"
  Sum/1 -> Gain2/1

== system node23_case_10kV_withLoad_v2/IBR4/IBR1输出电压正负序分离/k=0.4 ==
  u : Inport
  Gain1 : Gain  Gain=314.15926
  Gain2 : Gain  Gain=0.707
  Gain3 : Gain  Gain=314.15926
  Integrator : Integrator
  Integrator1 : Integrator
  Sum : Sum  Inputs=-+|
  Sum1 : Sum  Inputs=|+-
  u' : Outport
  qu' : Outport  Port=2
  wires:
  Gain1/1 -> Integrator/1
  Sum1/1 -> Gain1/1
  u/1 -> Sum/2
  Integrator/1 -> Integrator1/1, u'/1, Sum/1  "u'"
  Gain2/1 -> Sum1/1
  Integrator1/1 -> Gain3/1
  Gain3/1 -> qu'/1, Sum1/2  "qu'"
  Sum/1 -> Gain2/1

== system node23_case_10kV_withLoad_v2/IBR4/IBR1输出电流正负序分离/k=0.1 ==
  u : Inport
  Gain1 : Gain  Gain=314.15926
  Gain2 : Gain  Gain=0.707
  Gain3 : Gain  Gain=314.15926
  Integrator : Integrator
  Integrator1 : Integrator
  Sum : Sum  Inputs=-+|
  Sum1 : Sum  Inputs=|+-
  u' : Outport
  qu' : Outport  Port=2
  wires:
  Sum/1 -> Gain2/1
  Gain3/1 -> Sum1/2, qu'/1  "qu'"
  Integrator1/1 -> Gain3/1
  Gain2/1 -> Sum1/1
  Integrator/1 -> Sum/1, u'/1, Integrator1/1  "u'"
  u/1 -> Sum/2
  Sum1/1 -> Gain1/1
  Gain1/1 -> Integrator/1

== system node23_case_10kV_withLoad_v2/IBR4/IBR1输出电流正负序分离/k=0.4 ==
  u : Inport
  Gain1 : Gain  Gain=314.15926
  Gain2 : Gain  Gain=0.707
  Gain3 : Gain  Gain=314.15926
  Integrator : Integrator
  Integrator1 : Integrator
  Sum : Sum  Inputs=-+|
  Sum1 : Sum  Inputs=|+-
  u' : Outport
  qu' : Outport  Port=2
  wires:
  Sum/1 -> Gain2/1
  Gain3/1 -> Sum1/2, qu'/1  "qu'"
  Integrator1/1 -> Gain3/1
  Gain2/1 -> Sum1/1
  Integrator/1 -> Sum/1, u'/1, Integrator1/1  "u'"
  u/1 -> Sum/2
  Sum1/1 -> Gain1/1
  Gain1/1 -> Integrator/1

== matlab function node23_case_10kV_withLoad_v2/IBR-21/IBR1输出电压正负序分离/albe-dq ==
  data: valpha input; vd output; vbeta input; ph input; vq output
function [vd,vq] = fcn(valpha,vbeta,ph)
vd=cos(ph)*valpha+sin(ph)*vbeta;
vq=-sin(ph)*valpha+cos(ph)*vbeta;

== matlab function node23_case_10kV_withLoad_v2/IBR-21/IBR1输出电压正负序分离/alphabeta-dq 1 ==
  data: valpha input; vd output; vbeta input; ph input; vq output
function [vd,vq] = fcn(valpha,vbeta,ph)
vd=cos(ph)*valpha+sin(ph)*vbeta;
vq=-sin(ph)*valpha+cos(ph)*vbeta;

== matlab function node23_case_10kV_withLoad_v2/IBR-21/IBR1输出电流正负序分离/abc-alphabeta 1 ==
  data: va input; valpha output; vb input; vc input; vbeta output
function [valpha,vbeta] = fcn(va,vb,vc)
valpha=(2/3)*(1*va-1/2*vb-1/2*vc);
vbeta=(2/3)*(0*va+sqrt(3)/2*vb-sqrt(3)/2*vc);

== matlab function node23_case_10kV_withLoad_v2/IBR-21/IBR1输出电流正负序分离/albe-dq ==
  data: valpha input; vd output; vbeta input; ph input; vq output
function [vd,vq] = fcn(valpha,vbeta,ph)
vd=cos(ph)*valpha+sin(ph)*vbeta;
vq=-sin(ph)*valpha+cos(ph)*vbeta;

== matlab function node23_case_10kV_withLoad_v2/IBR-21/IBR1输出电流正负序分离/alphabeta-dq 1 ==
  data: valpha input; vd output; vbeta input; ph input; vq output
function [vd,vq] = fcn(valpha,vbeta,ph)
vd=cos(ph)*valpha+sin(ph)*vbeta;
vq=-sin(ph)*valpha+cos(ph)*vbeta;

== matlab function node23_case_10kV_withLoad_v2/IBR-21/IBR7 ==
  data: vcd_p input; Vc_p output; vcq_p input; vcd_n input; vcq_n input; Vc_n output; VUF output
function [Vc_p, Vc_n, VUF] = fcn(vcd_p, vcq_p, vcd_n, vcq_n)
Vc_p = sqrt(vcd_p^2 + vcq_p^2);
Vc_n = sqrt(vcd_n^2 + vcq_n^2);
VUF = Vc_n/Vc_p;

== matlab function node23_case_10kV_withLoad_v2/IBR-21/MATLAB Function1 ==
  data: u input; y output
function y = fcn(u)
y = rem(u,2*pi);

== matlab function node23_case_10kV_withLoad_v2/IBR-21/MATLAB Function4 ==
  data: ud input; ua output; uq input; ub output; ph input
function [ua,ub]= fcn(ud,uq,ph)
ua=ud*cos(ph)-uq*sin(ph)
ub=ud*sin(ph)+uq*cos(ph)

== matlab function node23_case_10kV_withLoad_v2/T_n1 ==
  data: ud input; Idp output; uq input; ub output; ph input
function [Idp,ub]= fcn(ud,uq,ph)
Idp=ud*cos(ph)+uq*sin(ph);
ub=-ud*sin(ph)+uq*cos(ph);

== matlab function node23_case_10kV_withLoad_v2/IBR-21/MATLAB Function5 ==
  data: ud input; ua output; uq input; ub output; ph input
function [ua,ub]= fcn(ud,uq,ph)
ua=ud*cos(ph)-uq*sin(ph);
ub=ud*sin(ph)+uq*cos(ph);

== matlab function node23_case_10kV_withLoad_v2/IBR-21/abc-alphabeta 10 ==
  data: va input; valpha output; vb input; vc input; vbeta output
function [valpha,vbeta] = fcn(va,vb,vc)
valpha=(2/3)*(1*va-1/2*vb-1/2*vc);
vbeta=(2/3)*(0*va+sqrt(3)/2*vb-sqrt(3)/2*vc);

== matlab function node23_case_10kV_withLoad_v2/IBR-21/albe-dq ==
  data: valpha input; vd output; vbeta input; ph input; vq output
function [vd,vq] = fcn(valpha,vbeta,ph)
vd=cos(ph)*valpha+sin(ph)*vbeta;
vq=-sin(ph)*valpha+cos(ph)*vbeta;

== matlab function node23_case_10kV_withLoad_v2/IBR-21/alphabeta-dq 9 ==
  data: valpha input; vd output; vbeta input; ph input; vq output
function [vd,vq] = fcn(valpha,vbeta,ph)
vd=cos(ph)*valpha+sin(ph)*vbeta;
vq=-sin(ph)*valpha+cos(ph)*vbeta;

== matlab function node23_case_10kV_withLoad_v2/IBR-21/dq轴功率计算 ==
  data: vd_p input; P1 output; vq_p input; vd_n input; vq_n input; id_p input; iq_p input; id_n input; iq_n input; Q1 output; P_p output; P_n output; Q_p output; Q_n output
function [P1, Q1, P_p, P_n, Q_p, Q_n] = fcn(vd_p, vq_p, vd_n, vq_n, id_p, iq_p, id_n, iq_n)
P_p = 1.5*(vd_p*id_p + vq_p*iq_p);
P_n = 1.5*(vd_n*id_n + vq_n*iq_n);
Q_p = 1.5*(vq_p*id_p - vd_p*iq_p);
Q_n = 1.5*(vq_n*id_n - vd_n*iq_n);
P1 = 1.5*(vd_p*id_p + vq_p*iq_p + vd_n*id_n + vq_n*iq_n);
Q1 = 1.5*(vq_p*id_p - vd_p*iq_p + vq_n*id_n - vd_n*iq_n);

%1.5倍

== matlab function node23_case_10kV_withLoad_v2/IBR-22/IBR1输出电压正负序分离/abc-alphabeta 1 ==
  data: va input; valpha output; vb input; vc input; vbeta output
function [valpha,vbeta] = fcn(va,vb,vc)
valpha=(2/3)*(1*va-1/2*vb-1/2*vc);
vbeta=(2/3)*(0*va+sqrt(3)/2*vb-sqrt(3)/2*vc);

== matlab function node23_case_10kV_withLoad_v2/IBR-22/IBR1输出电压正负序分离/albe-dq ==
  data: valpha input; vd output; vbeta input; ph input; vq output
function [vd,vq] = fcn(valpha,vbeta,ph)
vd=cos(ph)*valpha+sin(ph)*vbeta;
vq=-sin(ph)*valpha+cos(ph)*vbeta;

== matlab function node23_case_10kV_withLoad_v2/IBR-22/IBR1输出电压正负序分离/alphabeta-dq 1 ==
  data: valpha input; vd output; vbeta input; ph input; vq output
function [vd,vq] = fcn(valpha,vbeta,ph)
vd=cos(ph)*valpha+sin(ph)*vbeta;
vq=-sin(ph)*valpha+cos(ph)*vbeta;

== matlab function node23_case_10kV_withLoad_v2/IBR-22/IBR1输出电流正负序分离/abc-alphabeta 1 ==
  data: va input; valpha output; vb input; vc input; vbeta output
function [valpha,vbeta] = fcn(va,vb,vc)
valpha=(2/3)*(1*va-1/2*vb-1/2*vc);
vbeta=(2/3)*(0*va+sqrt(3)/2*vb-sqrt(3)/2*vc);

== matlab function node23_case_10kV_withLoad_v2/T_n7 ==
  data: ud input; Idp output; uq input; ub output; ph input
function [Idp,ub]= fcn(ud,uq,ph)
Idp=ud*cos(ph)+uq*sin(ph);
ub=-ud*sin(ph)+uq*cos(ph);

== matlab function node23_case_10kV_withLoad_v2/IBR-22/IBR1输出电流正负序分离/albe-dq ==
  data: valpha input; vd output; vbeta input; ph input; vq output
function [vd,vq] = fcn(valpha,vbeta,ph)
vd=cos(ph)*valpha+sin(ph)*vbeta;
vq=-sin(ph)*valpha+cos(ph)*vbeta;

== matlab function node23_case_10kV_withLoad_v2/IBR-22/IBR1输出电流正负序分离/alphabeta-dq 1 ==
  data: valpha input; vd output; vbeta input; ph input; vq output
function [vd,vq] = fcn(valpha,vbeta,ph)
vd=cos(ph)*valpha+sin(ph)*vbeta;
vq=-sin(ph)*valpha+cos(ph)*vbeta;

== matlab function node23_case_10kV_withLoad_v2/IBR-22/IBR7 ==
  data: vcd_p input; Vc_p output; vcq_p input; vcd_n input; vcq_n input; Vc_n output; VUF output
function [Vc_p, Vc_n, VUF] = fcn(vcd_p, vcq_p, vcd_n, vcq_n)
Vc_p = sqrt(vcd_p^2 + vcq_p^2);
Vc_n = sqrt(vcd_n^2 + vcq_n^2);
VUF = Vc_n/Vc_p;

== matlab function node23_case_10kV_withLoad_v2/IBR-22/MATLAB Function1 ==
  data: u input; y output
function y = fcn(u)
y = rem(u,2*pi);

== matlab function node23_case_10kV_withLoad_v2/IBR-22/MATLAB Function4 ==
  data: ud input; ua output; uq input; ub output; ph input
function [ua,ub]= fcn(ud,uq,ph)
ua=ud*cos(ph)-uq*sin(ph)
ub=ud*sin(ph)+uq*cos(ph)

== matlab function node23_case_10kV_withLoad_v2/IBR-22/MATLAB Function5 ==
  data: ud input; ua output; uq input; ub output; ph input
function [ua,ub]= fcn(ud,uq,ph)
ua=ud*cos(ph)-uq*sin(ph);
ub=ud*sin(ph)+uq*cos(ph);

== matlab function node23_case_10kV_withLoad_v2/IBR-22/abc-alphabeta 10 ==
  data: va input; valpha output; vb input; vc input; vbeta output
function [valpha,vbeta] = fcn(va,vb,vc)
valpha=(2/3)*(1*va-1/2*vb-1/2*vc);
vbeta=(2/3)*(0*va+sqrt(3)/2*vb-sqrt(3)/2*vc);

== matlab function node23_case_10kV_withLoad_v2/IBR-22/albe-dq ==
  data: valpha input; vd output; vbeta input; ph input; vq output
function [vd,vq] = fcn(valpha,vbeta,ph)
vd=cos(ph)*valpha+sin(ph)*vbeta;
vq=-sin(ph)*valpha+cos(ph)*vbeta;

== matlab function node23_case_10kV_withLoad_v2/IBR-22/alphabeta-dq 9 ==
  data: valpha input; vd output; vbeta input; ph input; vq output
function [vd,vq] = fcn(valpha,vbeta,ph)
vd=cos(ph)*valpha+sin(ph)*vbeta;
vq=-sin(ph)*valpha+cos(ph)*vbeta;

== matlab function node23_case_10kV_withLoad_v2/IBR-22/dq轴功率计算 ==
  data: vd_p input; P1 output; vq_p input; vd_n input; vq_n input; id_p input; iq_p input; id_n input; iq_n input; Q1 output; P_p output; P_n output; Q_p output; Q_n output
function [P1, Q1, P_p, P_n, Q_p, Q_n] = fcn(vd_p, vq_p, vd_n, vq_n, id_p, iq_p, id_n, iq_n)
P_p = 1.5*(vd_p*id_p + vq_p*iq_p);
P_n = 1.5*(vd_n*id_n + vq_n*iq_n);
Q_p = 1.5*(vq_p*id_p - vd_p*iq_p);
Q_n = 1.5*(vq_n*id_n - vd_n*iq_n);
P1 = 1.5*(vd_p*id_p + vq_p*iq_p + vd_n*id_n + vq_n*iq_n);
Q1 = 1.5*(vq_p*id_p - vd_p*iq_p + vq_n*id_n - vd_n*iq_n);

%1.5倍

== matlab function node23_case_10kV_withLoad_v2/IBR-10/IBR1输出电压正负序分离/abc-alphabeta 1 ==
  data: va input; valpha output; vb input; vc input; vbeta output
function [valpha,vbeta] = fcn(va,vb,vc)
valpha=(2/3)*(1*va-1/2*vb-1/2*vc);
vbeta=(2/3)*(0*va+sqrt(3)/2*vb-sqrt(3)/2*vc);

== matlab function node23_case_10kV_withLoad_v2/IBR-23/IBR1输出电压正负序分离/abc-alphabeta 1 ==
  data: va input; valpha output; vb input; vc input; vbeta output
function [valpha,vbeta] = fcn(va,vb,vc)
valpha=(2/3)*(1*va-1/2*vb-1/2*vc);
vbeta=(2/3)*(0*va+sqrt(3)/2*vb-sqrt(3)/2*vc);

== matlab function node23_case_10kV_withLoad_v2/IBR-23/IBR1输出电压正负序分离/albe-dq ==
  data: valpha input; vd output; vbeta input; ph input; vq output
function [vd,vq] = fcn(valpha,vbeta,ph)
vd=cos(ph)*valpha+sin(ph)*vbeta;
vq=-sin(ph)*valpha+cos(ph)*vbeta;

== matlab function node23_case_10kV_withLoad_v2/IBR-23/IBR1输出电压正负序分离/alphabeta-dq 1 ==
  data: valpha input; vd output; vbeta input; ph input; vq output
function [vd,vq] = fcn(valpha,vbeta,ph)
vd=cos(ph)*valpha+sin(ph)*vbeta;
vq=-sin(ph)*valpha+cos(ph)*vbeta;

== matlab function node23_case_10kV_withLoad_v2/IBR-23/IBR1输出电流正负序分离/abc-alphabeta 1 ==
  data: va input; valpha output; vb input; vc input; vbeta output
function [valpha,vbeta] = fcn(va,vb,vc)
valpha=(2/3)*(1*va-1/2*vb-1/2*vc);
vbeta=(2/3)*(0*va+sqrt(3)/2*vb-sqrt(3)/2*vc);

== matlab function node23_case_10kV_withLoad_v2/IBR-23/IBR1输出电流正负序分离/albe-dq ==
  data: valpha input; vd output; vbeta input; ph input; vq output
function [vd,vq] = fcn(valpha,vbeta,ph)
vd=cos(ph)*valpha+sin(ph)*vbeta;
vq=-sin(ph)*valpha+cos(ph)*vbeta;

== matlab function node23_case_10kV_withLoad_v2/IBR-23/IBR1输出电流正负序分离/alphabeta-dq 1 ==
  data: valpha input; vd output; vbeta input; ph input; vq output
function [vd,vq] = fcn(valpha,vbeta,ph)
vd=cos(ph)*valpha+sin(ph)*vbeta;
vq=-sin(ph)*valpha+cos(ph)*vbeta;

== matlab function node23_case_10kV_withLoad_v2/IBR-23/IBR7 ==
  data: vcd_p input; Vc_p output; vcq_p input; vcd_n input; vcq_n input; Vc_n output; VUF output
function [Vc_p, Vc_n, VUF] = fcn(vcd_p, vcq_p, vcd_n, vcq_n)
Vc_p = sqrt(vcd_p^2 + vcq_p^2);
Vc_n = sqrt(vcd_n^2 + vcq_n^2);
VUF = Vc_n/Vc_p;

== matlab function node23_case_10kV_withLoad_v2/IBR-23/MATLAB Function1 ==
  data: u input; y output
function y = fcn(u)
y = rem(u,2*pi);

== matlab function node23_case_10kV_withLoad_v2/IBR-23/MATLAB Function4 ==
  data: ud input; ua output; uq input; ub output; ph input
function [ua,ub]= fcn(ud,uq,ph)
ua=ud*cos(ph)-uq*sin(ph)
ub=ud*sin(ph)+uq*cos(ph)

== matlab function node23_case_10kV_withLoad_v2/IBR4/MATLAB Function1 ==
  data: u input; y output
function y = fcn(u)
y = rem(u,2*pi);

== matlab function node23_case_10kV_withLoad_v2/IBR-23/MATLAB Function5 ==
  data: ud input; ua output; uq input; ub output; ph input
function [ua,ub]= fcn(ud,uq,ph)
ua=ud*cos(ph)-uq*sin(ph);
ub=ud*sin(ph)+uq*cos(ph);

== matlab function node23_case_10kV_withLoad_v2/IBR-23/abc-alphabeta 10 ==
  data: va input; valpha output; vb input; vc input; vbeta output
function [valpha,vbeta] = fcn(va,vb,vc)
valpha=(2/3)*(1*va-1/2*vb-1/2*vc);
vbeta=(2/3)*(0*va+sqrt(3)/2*vb-sqrt(3)/2*vc);

== matlab function node23_case_10kV_withLoad_v2/IBR-23/albe-dq ==
  data: valpha input; vd output; vbeta input; ph input; vq output
function [vd,vq] = fcn(valpha,vbeta,ph)
vd=cos(ph)*valpha+sin(ph)*vbeta;
vq=-sin(ph)*valpha+cos(ph)*vbeta;

== matlab function node23_case_10kV_withLoad_v2/IBR-23/alphabeta-dq 9 ==
  data: valpha input; vd output; vbeta input; ph input; vq output
function [vd,vq] = fcn(valpha,vbeta,ph)
vd=cos(ph)*valpha+sin(ph)*vbeta;
vq=-sin(ph)*valpha+cos(ph)*vbeta;

== matlab function node23_case_10kV_withLoad_v2/IBR-23/dq轴功率计算 ==
  data: vd_p input; P1 output; vq_p input; vd_n input; vq_n input; id_p input; iq_p input; id_n input; iq_n input; Q1 output; P_p output; P_n output; Q_p output; Q_n output
function [P1, Q1, P_p, P_n, Q_p, Q_n] = fcn(vd_p, vq_p, vd_n, vq_n, id_p, iq_p, id_n, iq_n)
P_p = 1.5*(vd_p*id_p + vq_p*iq_p);
P_n = 1.5*(vd_n*id_n + vq_n*iq_n);
Q_p = 1.5*(vq_p*id_p - vd_p*iq_p);
Q_n = 1.5*(vq_n*id_n - vd_n*iq_n);
P1 = 1.5*(vd_p*id_p + vq_p*iq_p + vd_n*id_n + vq_n*iq_n);
Q1 = 1.5*(vq_p*id_p - vd_p*iq_p + vq_n*id_n - vd_n*iq_n);

%1.5倍

== matlab function node23_case_10kV_withLoad_v2/IBR4/MATLAB Function2 ==
  data: u input; y output
function y = fcn(u)
y = rem(u,2*pi);

== matlab function node23_case_10kV_withLoad_v2/IBR-8/MATLAB Function2 ==
  data: u input; y output
function y = fcn(u)
y = rem(u,2*pi);

== matlab function node23_case_10kV_withLoad_v2/IBR4/abc-alphabeta 10 ==
  data: va input; valpha output; vb input; vc input; vbeta output
function [valpha,vbeta] = fcn(va,vb,vc)
valpha=(2/3)*(1*va-1/2*vb-1/2*vc);
vbeta=(2/3)*(0*va+sqrt(3)/2*vb-sqrt(3)/2*vc);

== matlab function node23_case_10kV_withLoad_v2/IBR-10/MATLAB Function2 ==
  data: u input; y output
function y = fcn(u)
y = rem(u,2*pi);

== matlab function node23_case_10kV_withLoad_v2/IBR-11/MATLAB Function2 ==
  data: u input; y output
function y = fcn(u)
y = rem(u,2*pi);

== matlab function node23_case_10kV_withLoad_v2/IBR-12/MATLAB Function2 ==
  data: u input; y output
function y = fcn(u)
y = rem(u,2*pi);

== matlab function node23_case_10kV_withLoad_v2/IBR-16/MATLAB Function2 ==
  data: u input; y output
function y = fcn(u)
y = rem(u,2*pi);

== matlab function node23_case_10kV_withLoad_v2/IBR-21/MATLAB Function2 ==
  data: u input; y output
function y = fcn(u)
y = rem(u,2*pi);

== matlab function node23_case_10kV_withLoad_v2/IBR-22/MATLAB Function2 ==
  data: u input; y output
function y = fcn(u)
y = rem(u,2*pi);

== matlab function node23_case_10kV_withLoad_v2/IBR-23/MATLAB Function2 ==
  data: u input; y output
function y = fcn(u)
y = rem(u,2*pi);

== matlab function node23_case_10kV_withLoad_v2/IBR1输出电压正负序分离/abc-alphabeta 1 ==
  data: va input; valpha output; vb input; vc input; vbeta output
function [valpha,vbeta] = fcn(va,vb,vc)
valpha=(2/3)*(1*va-1/2*vb-1/2*vc);
vbeta=(2/3)*(0*va+sqrt(3)/2*vb-sqrt(3)/2*vc);

== matlab function node23_case_10kV_withLoad_v2/IBR1输出电压正负序分离/albe-dq ==
  data: valpha input; vd output; vbeta input; ph input; vq output
function [vd,vq] = fcn(valpha,vbeta,ph)
vd=cos(ph)*valpha+sin(ph)*vbeta;
vq=-sin(ph)*valpha+cos(ph)*vbeta;

== matlab function node23_case_10kV_withLoad_v2/IBR1输出电压正负序分离/alphabeta-dq 1 ==
  data: valpha input; vd output; vbeta input; ph input; vq output
function [vd,vq] = fcn(valpha,vbeta,ph)
vd=cos(ph)*valpha+sin(ph)*vbeta;
vq=-sin(ph)*valpha+cos(ph)*vbeta;

== matlab function node23_case_10kV_withLoad_v2/IBR2 ==
  data: vcd_p input; Vc_p output; vcq_p input; vcd_n input; vcq_n input; Vc_n output; VUF output
function [Vc_p, Vc_n, VUF] = fcn(vcd_p, vcq_p, vcd_n, vcq_n)
Vc_p = sqrt(vcd_p^2 + vcq_p^2);
Vc_n = sqrt(vcd_n^2 + vcq_n^2);
VUF = Vc_n/Vc_p;

== matlab function node23_case_10kV_withLoad_v2/IBR1 ==
  data: vcd_p input; Vc_p output; vcq_p input; vcd_n input; vcq_n input; Vc_n output; VUF output
function [Vc_p, Vc_n, VUF] = fcn(vcd_p, vcq_p, vcd_n, vcq_n)
Vc_p = sqrt(vcd_p^2 + vcq_p^2);
Vc_n = sqrt(vcd_n^2 + vcq_n^2);
VUF = Vc_n/Vc_p;

== matlab function node23_case_10kV_withLoad_v2/IBR4/alphabeta-dq 9 ==
  data: valpha input; vd output; vbeta input; ph input; vq output
function [vd,vq] = fcn(valpha,vbeta,ph)
vd=cos(ph)*valpha+sin(ph)*vbeta;
vq=-sin(ph)*valpha+cos(ph)*vbeta;

== matlab function node23_case_10kV_withLoad_v2/IBR1输出电压正负序分离1/abc-alphabeta 1 ==
  data: va input; valpha output; vb input; vc input; vbeta output
function [valpha,vbeta] = fcn(va,vb,vc)
valpha=(2/3)*(1*va-1/2*vb-1/2*vc);
vbeta=(2/3)*(0*va+sqrt(3)/2*vb-sqrt(3)/2*vc);

== matlab function node23_case_10kV_withLoad_v2/IBR1输出电压正负序分离1/albe-dq ==
  data: valpha input; vd output; vbeta input; ph input; vq output
function [vd,vq] = fcn(valpha,vbeta,ph)
vd=cos(ph)*valpha+sin(ph)*vbeta;
vq=-sin(ph)*valpha+cos(ph)*vbeta;

== matlab function node23_case_10kV_withLoad_v2/IBR1输出电压正负序分离1/alphabeta-dq 1 ==
  data: valpha input; vd output; vbeta input; ph input; vq output
function [vd,vq] = fcn(valpha,vbeta,ph)
vd=cos(ph)*valpha+sin(ph)*vbeta;
vq=-sin(ph)*valpha+cos(ph)*vbeta;

== matlab function node23_case_10kV_withLoad_v2/IBR-10/IBR1输出电压正负序分离/albe-dq ==
  data: valpha input; vd output; vbeta input; ph input; vq output
function [vd,vq] = fcn(valpha,vbeta,ph)
vd=cos(ph)*valpha+sin(ph)*vbeta;
vq=-sin(ph)*valpha+cos(ph)*vbeta;
